simulink model "MIT"  (R2021b)
settings: Solver=VariableStepAuto  StartTime=0.0  StopTime=6000  RelTol=1e-4
values from neighbouring files (symbols this model uses):
  den_real = [1, a1_number, a2_number]    [Main.m]
  num_real = [R2/(tau1*tau2)]    [Main.m]
  period = set_time * 15*2    (= 3000)    [Main.m]
undefined symbols (not defined in the file or in its folder): den_des, num_des
libraries: dspstat3 x10, dspsrcs4 x1
settings Model: Creator=mahdi  LastModifiedBy=mahdi

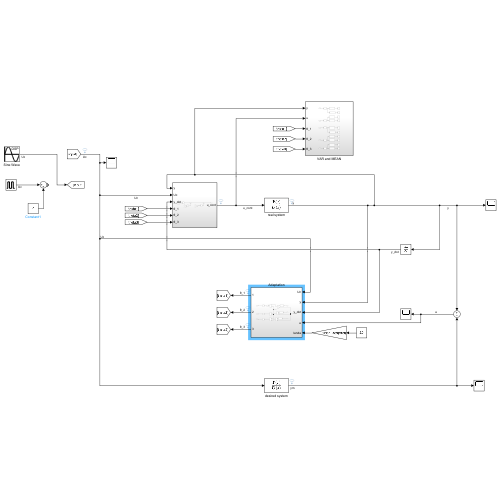
[thumbnail: Simulink's stored preview of the top-level diagram]
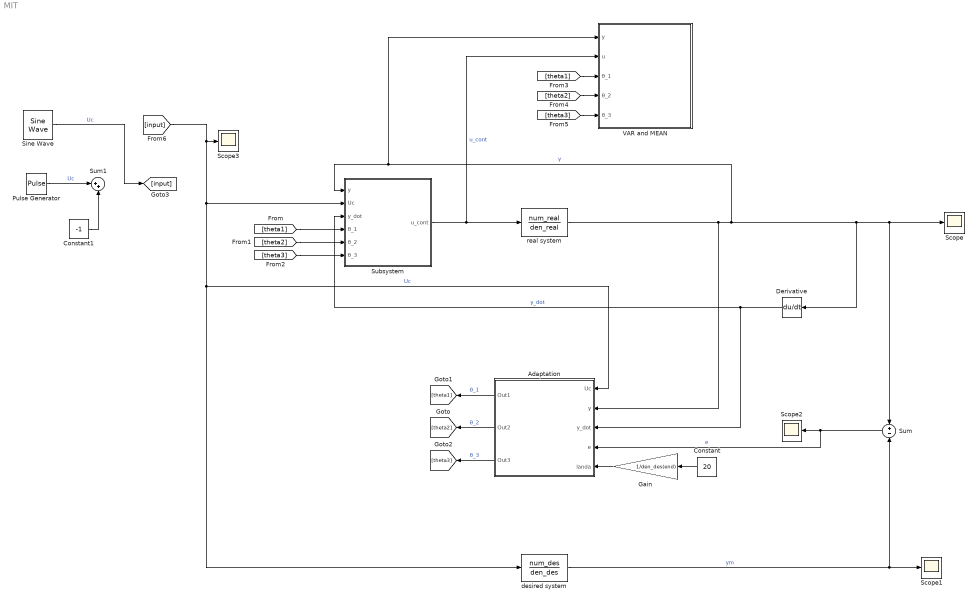
== system MIT ==
  Adaptation : Subsystem
  Constant : Constant  Value=20
  Constant1 : Constant  Value=-1
  Derivative : Derivative
  Gain : Gain  Gain=1/den_des(end)
  Pulse Generator : DiscretePulseGenerator  PulseType=Time based  Amplitude=2  Period=period  PulseWidth=50
  Scope{,1..3} (4 alike) : Scope
  Sine Wave : dspsrcs4/Sine Wave  Amplitude=1  Frequency=0.001  Phase=0  SampleMode=Continuous  OutComplex=Real  CompMethod=Trigonometric fcn  TableSize=Speed  SampleTime=0  SamplesPerFrame=1  ResetState=Restart at time zero  OutputFrames=off  dataType=double  wordLen=16  udDataType=sfix(16)  fracBitsMode=Best precision  numFracBits=15  OutDataTypeStr=double  LastOutDataTypeStr=double
  Subsystem : Subsystem
  Sum : Sum  Inputs=+|-
  Sum1 : Sum  Inputs=|++
  VAR and MEAN : Subsystem
  desired system : TransferFcn  Numerator=num_des  Denominator=den_des
  real system : TransferFcn  Numerator=num_real  Denominator=den_real
  wires:
  real system/1 -> VAR and MEAN/1(y), Subsystem/1(y), Scope/1, Sum/1, Derivative/1, Adaptation/2(y)  "y"
  [input] -> Adaptation/1(Uc), desired system/1, Subsystem/2(Uc), Scope3/1  "Uc"
  desired system/1 -> Sum/2, Scope1/1  "ym"
  Derivative/1 -> Subsystem/3(y_dot), Adaptation/3(y_dot)  "y_dot"
  Sum/1 -> Adaptation/4(e), Scope2/1  "e"
  Adaptation/1(Out1) -> [theta1]  "θ_1"
  Adaptation/2(Out2) -> [theta2]  "θ_2"
  Adaptation/3(Out3) -> [theta3]  "θ_3"
  Gain/1 -> Adaptation/5(landa)
  Constant/1 -> Gain/1
  Pulse Generator/1 -> Sum1/1  "Uc"
  Constant1/1 -> Sum1/2
  [theta1] -> Subsystem/4(θ_1)
  [theta2] -> Subsystem/5(θ_2)
  [theta3] -> Subsystem/6(θ_3)
  Subsystem/1(u_cont) -> VAR and MEAN/2(u), real system/1  "u_cont"
  [theta2] -> VAR and MEAN/4(θ_2)
  [theta3] -> VAR and MEAN/5(θ_3)
  [theta1] -> VAR and MEAN/3(θ_1)
  Sine Wave/1 -> [input]  "Uc"

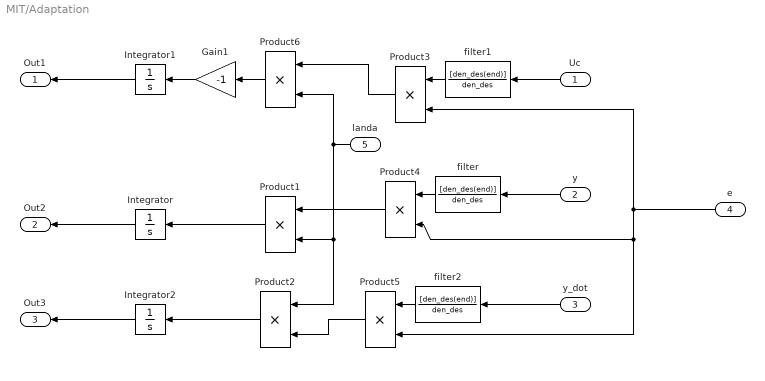
== system MIT/Adaptation ==
  Uc : Inport
  y : Inport  Port=2
  y_dot : Inport  Port=3
  e : Inport  Port=4
  landa : Inport  Port=5
  Gain1 : Gain  Gain=-1
  Integrator : Integrator
  Integrator1 : Integrator
  Integrator2 : Integrator
  Product{1..6} (6 alike) : Product
  filter : TransferFcn  Numerator=[den_des(end)]  Denominator=den_des
  filter1 : TransferFcn  Numerator=[den_des(end)]  Denominator=den_des
  filter2 : TransferFcn  Numerator=[den_des(end)]  Denominator=den_des
  Out1 : Outport
  Out2 : Outport  Port=2
  Out3 : Outport  Port=3
  wires:
  filter1/1 -> Product3/1
  Integrator1/1 -> Out1/1
  Integrator2/1 -> Out3/1
  filter2/1 -> Product5/1
  Integrator/1 -> Out2/1
  Product1/1 -> Integrator/1
  Product5/1 -> Product2/2
  Product2/1 -> Integrator2/1
  Product4/1 -> Product1/1
  filter/1 -> Product4/1
  Uc/1 -> filter1/1
  Gain1/1 -> Integrator1/1
  y/1 -> filter/1
  y_dot/1 -> filter2/1
  e/1 -> Product3/2, Product4/2, Product5/2
  Product3/1 -> Product6/1
  Product6/1 -> Gain1/1
  landa/1 -> Product2/1, Product1/2, Product6/2

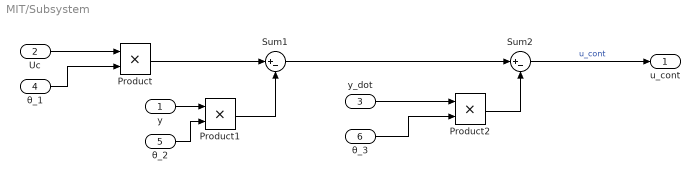
== system MIT/Subsystem ==
  y : Inport
  Uc : Inport  Port=2
  y_dot : Inport  Port=3
  θ_1 : Inport  Port=4
  θ_2 : Inport  Port=5
  θ_3 : Inport  Port=6
  Product : Product
  Product1 : Product
  Product2 : Product
  Sum1 : Sum  Inputs=|+-
  Sum2 : Sum  Inputs=|+-
  u_cont : Outport
  wires:
  y_dot/1 -> Product2/1
  Product1/1 -> Sum1/2
  Product2/1 -> Sum2/2
  θ_1/1 -> Product/2
  Sum1/1 -> Sum2/1
  Product/1 -> Sum1/1
  θ_2/1 -> Product1/2
  Sum2/1 -> u_cont/1  "u_cont"
  y/1 -> Product1/1
  θ_3/1 -> Product2/2
  Uc/1 -> Product/1

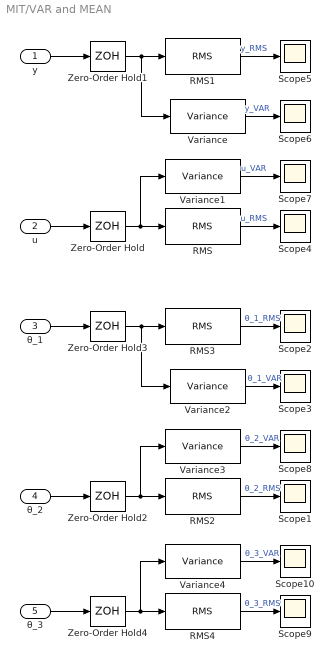
== system MIT/VAR and MEAN ==
  y : Inport
  u : Inport  Port=2
  θ_1 : Inport  Port=3
  θ_2 : Inport  Port=4
  θ_3 : Inport  Port=5
  RMS{,1..4} (5 alike) : dspstat3/RMS  run=off  directionMode=Each column  dimension=1  InputProcessing=Columns as channels (frame based)  reset_popup=None
  Scope{1..10} (10 alike) : Scope
  Variance{,1..4} (5 alike) : dspstat3/Variance  run=on  InputProcessing=Columns as channels (frame based)  reset_popup=None  directionMode=Each column  dimension=1  roiEnable=off  roiType=Rectangles  roiPortion=Entire ROI  roiOutput=Individual statistics for each ROI  roiFlag=off  roundingMode=Floor  overflowMode=off
  Zero-Order Hold{,1..4} (5 alike) : ZeroOrderHold
  wires:
  Zero-Order Hold1/1 -> Variance/1, RMS1/1
  Zero-Order Hold/1 -> Variance1/1, RMS/1
  Variance1/1 -> Scope7/1  "u_VAR"
  y/1 -> Zero-Order Hold1/1
  RMS1/1 -> Scope5/1  "y_RMS"
  u/1 -> Zero-Order Hold/1
  RMS/1 -> Scope4/1  "u_RMS"
  Variance/1 -> Scope6/1  "y_VAR"
  θ_2/1 -> Zero-Order Hold2/1
  Variance2/1 -> Scope3/1  "θ_1_VAR"
  RMS2/1 -> Scope1/1  "θ_2_RMS"
  RMS3/1 -> Scope2/1  "θ_1_RMS"
  Zero-Order Hold3/1 -> Variance2/1, RMS3/1
  Zero-Order Hold2/1 -> Variance3/1, RMS2/1
  Variance3/1 -> Scope8/1  "θ_2_VAR"
  θ_1/1 -> Zero-Order Hold3/1
  Variance4/1 -> Scope10/1  "θ_3_VAR"
  RMS4/1 -> Scope9/1  "θ_3_RMS"
  Zero-Order Hold4/1 -> Variance4/1, RMS4/1
  θ_3/1 -> Zero-Order Hold4/1
